simulink model "Basic_Communication_System"  (Simulink 9.3)
settings: Solver=ode45  StartTime=0.0  StopTime=inf  RelTol=1e-3  EnableMultiTasking=on
undefined symbols (not defined in the file or in its folder): gcbh, rcfiltgaincompat
libraries: commutil2 x2, commfilt2 x2, commdigbbndam3 x2, dspquant2 x2, commchan3 x1, dsparch4 x1, commsink2 x1
settings Model: Creator=Jinwoo Kim  LastModifiedBy=hwanju
settings DataIOCC: LimitDataPoints=on
settings OptimizationCC: ExpressionDepthLimit=2147483647  InitFltsAndDblsToZero=on
settings DebuggingCC: SaveWithParameterizedLinksMsg=none  SignalResolutionControl=TryResolveAllWithWarning  SolverPrmCheckMsg=warning  MultiTaskDSMMsg=warning  MultiTaskCondExecSysMsg=none  StateNameClashWarn=warning  SFExecutionAtInitializationDiag=warning
settings GRTTargetCC: TargetFcnLib=ansi_tfl_tmw.mat  GeneratePreprocessorConditionals=Disable all

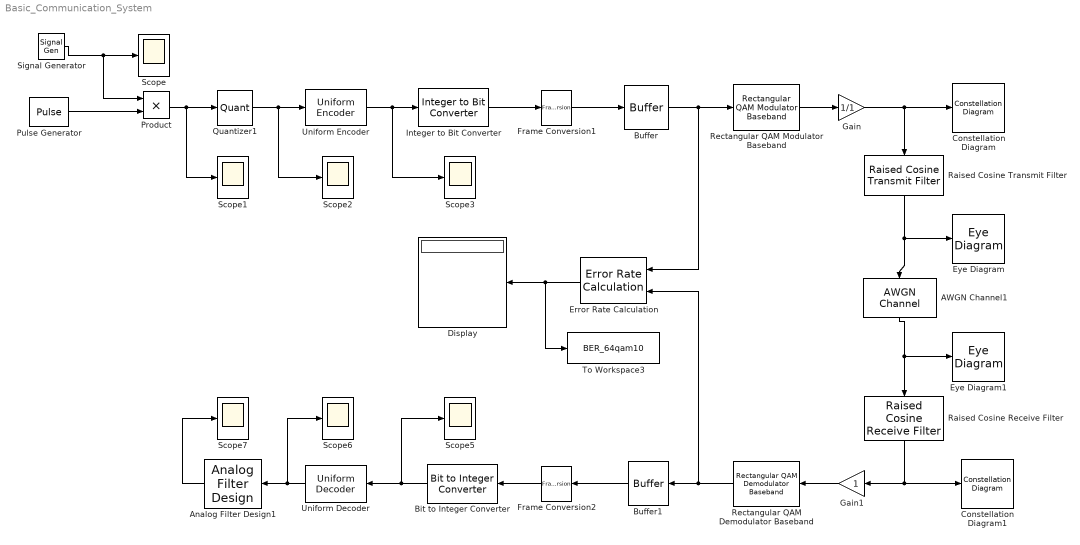
== system Basic_Communication_System ==
  AWGN Channel1 : commchan3/AWGN Channel  InputProcessing=Columns as channels (frame based)  seed=84  noiseMode="Signal to noise ratio  (Eb/No)"  EbNodB=1  EsNodB=10  SNRdB=30  bitsPerSym=4  Ps=1  Tsym=1/6e4*4/8  variance=1
      settings: SourceProductName=Communications Toolbox
  Analog Filter Design1 : dsparch4/Analog Filter Design  method=Butterworth  filttype=Lowpass  N=18  Wlo=4*pi*1e3  Whi=80  Rp=2  Rs=40
  Bit to Integer Converter : commutil2/Bit to Integer Converter  nbits=6  bitOrder=MSB first  signedOutputValues=Unsigned  outDtype=uint8  outDtypeSigned=Inherit via internal rule
      settings: SourceProductName=Communications Toolbox
  Buffer : Buffer  N=4
  Buffer1 : Buffer  N=6
  Constellation Diagram : ConstellationDiagram
  Constellation Diagram1 : ConstellationDiagram
  Display : Display
  Error Rate Calculation : commsink2/Error Rate Calculation  N=4*4*2  st_delay=0  cp_mode=Entire frame  subframe=[]  PMode=Port  WsName=ErrorVec  RsMode2=off  stop=off  numErr=100  maxBits=1e6
      settings: SourceProductName=Communications Toolbox
  Eye Diagram : EyeDiagram
  Eye Diagram1 : EyeDiagram
  Frame Conversion1 : FrameConversion
  Frame Conversion2 : FrameConversion  OutFrame=Sample-based
  Gain : Gain  Gain=1/1
  Gain1 : Gain
  Integer to Bit Converter : commutil2/Integer to Bit Converter  nbits=6  signedInputValues=Unsigned  bitOrder=MSB first  outDtype=double
      settings: SourceProductName=Communications Toolbox
  Product : Product  RndMeth=Zero
  Pulse Generator : DiscretePulseGenerator  PulseType=Time based  Period=1/1e4  PulseWidth=0.025
  Quantizer1 : Quantizer  QuantizationInterval=10/32  LinearizeAsGain=off  SampleTime=1/1e4
  Raised Cosine Receive Filter : commfilt2/Raised Cosine Receive Filter  filtType=Square root  R=0.25  filtSpan=2*4  N=8  downFactor=8  downOffset=0  filterGain=rcfiltgaincompat(gcbh)  InputProcessing=Columns as channels (frame based)  RateOptions=Enforce single-rate processing  framing=Mute  checkCoeff=off  variableName=rcRxFilt  currentFiltSpan=2*4  D=(2*4)/2  inputOffset=0  sampMode=Mute  saveAsFlag=0  rateMode=Downsampling  checkGain=Normalized  launchFVT=off  roundingMode=Floor  overflowMode=off  coeffDataTypeStr=Inherit: Same word length as input  coeffMin=[]  coeffMax=[]  coeffLastDataTypeStr=Inherit: Same word length as input  accumDataTypeStr=Inherit: Same as product output  accumLastDataTypeStr=Inherit: Same as product output  outputDataTypeStr=Inherit: Same as accumulator  outputMin=[]  outputMax=[]  outputLastDataTypeStr=Inherit: Same as accumulator
      settings: SourceProductName=Communications Toolbox
  Raised Cosine Transmit Filter : commfilt2/Raised Cosine Transmit Filter  filtType=Square root  R=1  filtSpan=2*4  N=8  filterGain=rcfiltgaincompat(gcbh)  InputProcessing=Columns as channels (frame based)  RateOptions=Enforce single-rate processing  framing=Mute  checkCoeff=off  variableName=rcTxFilt  checkGain=Normalized  sampMode=Mute  saveAsFlag=0  currentFiltSpan=2*4  D=(2*4)/2  launchFVT=off  roundingMode=Floor  overflowMode=off  coeffDataTypeStr=Inherit: Same word length as input  coeffMin=[]  coeffMax=[]  coeffLastDataTypeStr=Inherit: Same word length as input  outputDataTypeStr=Inherit: Same as accumulator  outputMin=[]  outputMax=[]  outputLastDataTypeStr=Inherit: Same as accumulator
      settings: SourceProductName=Communications Toolbox
  Rectangular QAM Demodulator Baseband : commdigbbndam3/Rectangular QAM Demodulator Baseband  M=2^4  OutType=Bit  DecType=Hard decision  VarSource=Dialog  Variance=1  Dec=Gray  Mapping=[0:15]  PowType=Min. distance between symbols  MinDist=2  AvgPow=1  PeakPow=1  Ph=0  outDtype1=double  outDtype2=double  derotateFactorWordLen=16  derotateFactorDataTypeStr=Inherit: Same word length as input  derotateFactorLastDataTypeStr=Inherit: Same word length as input  denormFactorWordLen=16  denormFactorDataTypeStr=Inherit: Same word length as input  denormFactorLastDataTypeStr=Inherit: Same word length as input  prodOutWordLen=32  prodOutOverflowMode=Wrap  prodOutRoundingMode=Floor  prodOutOvFlMode=off  prodOutOvFlModeLastStrValue=off  sumWordLen=32
      settings: SourceProductName=Communications Toolbox
  Rectangular QAM Modulator Baseband : commdigbbndam3/Rectangular QAM Modulator Baseband  M=2^4  InType=Bit  Enc=Gray  Mapping=[0:15]  PowType=Min. distance between symbols  MinDist=2  AvgPow=1  PeakPow=1  Ph=0  outDtype=double  outWordLen=16  outUDDataType=sfix(16)  outFracLenMode=Best precision  outFracLen=15  outDataTypeStr=double  outLastDataTypeStr=double
      settings: SourceProductName=Communications Toolbox
  Scope{,1..3,5..7} (7 alike) : Scope
  Signal Generator : SignalGenerator  Amplitude=10  Frequency=1e3
  To Workspace3 : ToWorkspace  VariableName=BER_64qam10  SampleTime=-1
      settings: MaxDataPoints=1
  Uniform Decoder : dspquant2/Uniform Decoder  peak=10  bits=6  overflowMode=Saturate  otype=Double
      settings: SourceProductName=DSP System Toolbox  SourceProductBaseCode=DS
  Uniform Encoder : dspquant2/Uniform Encoder  peak=10  bits=6  otype=Unsigned integer
      settings: SourceProductName=DSP System Toolbox
  wires:
  Signal Generator/1 -> Scope/1, Product/1
  Product/1 -> Scope1/1, Quantizer1/1
  Pulse Generator/1 -> Product/2
  AWGN Channel1/1 -> Eye Diagram1/1, Raised Cosine Receive Filter/1
  Uniform Decoder/1 -> Analog Filter Design1/1, Scope6/1
  Analog Filter Design1/1 -> Scope7/1
  Error Rate Calculation/1 -> To Workspace3/1, Display/1
  Bit to Integer Converter/1 -> Uniform Decoder/1, Scope5/1
  Rectangular QAM Demodulator Baseband/1 -> Error Rate Calculation/2, Buffer1/1
  Integer to Bit Converter/1 -> Frame Conversion1/1
  Quantizer1/1 -> Scope2/1, Uniform Encoder/1
  Buffer/1 -> Error Rate Calculation/1, Rectangular QAM Modulator Baseband/1
  Frame Conversion1/1 -> Buffer/1
  Buffer1/1 -> Frame Conversion2/1
  Uniform Encoder/1 -> Scope3/1, Integer to Bit Converter/1
  Rectangular QAM Modulator Baseband/1 -> Gain/1
  Frame Conversion2/1 -> Bit to Integer Converter/1
  Gain/1 -> Constellation Diagram/1, Raised Cosine Transmit Filter/1
  Gain1/1 -> Rectangular QAM Demodulator Baseband/1
  Raised Cosine Transmit Filter/1 -> Eye Diagram/1, AWGN Channel1/1
  Raised Cosine Receive Filter/1 -> Constellation Diagram1/1, Gain1/1
